simulink library "NI_Board_AO"  (Simulink 7.8)
settings: Solver=ode45  StartTime=0.0  StopTime=10.0  RelTol=1e-3
settings Model: Creator=Administrator  LastModifiedBy=Administrator

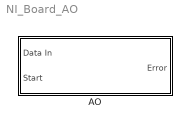
== system NI_Board_AO ==
  AO : Subsystem  mask(Analog Output v1){nCon=0, nDev=1, nChan=[1], nMax=10, nMin=-10, nSample=Voltage, nReserve=0}
      mask prompts: nCon "Control ID"; nDev "Dev ID"; nChan "Channel ID"; nMax "Maximum Value"; nMin "Minimum Value"; nSample "Mode"; nReserve "Reserve"
      mask help:
      | 模块用于 AO 数据的输出
      |
      | Data In
      | 输出到相应Channel的数据，维度与Channel对应
      |
      | Start
      | 当給值 1 时，相应通道做输出动作
      |
      | Error
      | 返回底层支持模块运行状态，不是 0 则出错
      |
      | Control ID
      | 用于标识不同的模块
      |
      | Dev ID
      | 用于标识通道位于哪一个板卡上，
      | 当使用 NI 数据采集系列板卡时，在下位机成功安装nidaqmx系列驱动后
      | 可通过命令行执行 nilsdev 查看，如果不在模块下拉序列中，可修改，
      | 修改方法参见 《NI board set.docx》
      |
      | Channel ID
      | 需要输出的ao通道号，可单一或者多个通过号同时输出
      | 单一通道时直接给值即可，如输出通道 2 ，可给值 2
      | 多个通道同时输出时，如输出通道 1 3 9，可给值 [1 3 9]
      | 通道号应小于 100
      |
      | Mode
      | 可选择输出方式，电压或电流
      | 不支持同一板卡不同通道采用不同输出方式
      mask init:
      | displayblock=sprintf('Control ID:%d\nDev:%d',nCon-1, nDev);
      mask StyleString: popup(0|1|2|3|4|5|6|7|8|9|10|11|12|13|14|15),popup(1|2|3|4|5|6|7|8|9|10|11|12|13|14|15|16|17|18|19|20|21|22|23|24|25|26|27|28|29|30|31|32),edit,edit,edit,popup(Voltage|Current),edit
      mask Display: disp(displayblock);

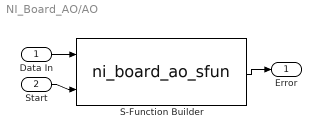
== system NI_Board_AO/AO ==
  Data In : Inport
  Start : Inport  Port=2
  S-Function Builder : S-Function  InitFcn=try, set_param(gcb,'FunctionName','ni_board_ao_sfun'), end  FunctionName=ni_board_ao_sfun  Parameters=1,1,1,1,1,1,1  WizardData=DataTag0  EnableBusSupport=off  mask(S-Function Builder){}
      mask help: Simulink:masks:SFunctionBuilder_MD
      mask init:
      | val = [[.9  0.75 0.75 1 1 .9 .9 1]',[1 1 0.75 0.75 .9 .9 1 .9]'];try , sys = get_param(gcb,'SfunBuilderFcnName');if isempty(sys), sys = get_param(gcb,'FunctionName'); end,catch, sys = get_param(gcb,'FunctionName'); end
      settings: CopyFcn=set_param(gcbh,'LinkStatus','none')  PreSaveFcn=try, set_param(gcb,'FunctionName','ni_board_ao_sfun'), end  OpenFcn=sfunctionwizard(gcbh)
      mask Display: plot(val(:,1),val(:,2)),disp(sys), port_label('input',1,'u0'), port_label('input',2,'u1'), port_label('output',1,'y0')
  Error : Outport
  wires:
  Start/1 -> S-Function Builder/2
  S-Function Builder/1 -> Error/1
  Data In/1 -> S-Function Builder/1
